simulink model "Isooffboard_SSC"  (R2026a)
settings: Solver=VariableStepAuto  StopTime=0.05
undefined symbols (not defined in the file): V_ref_isolated
libraries: fl_lib x73, nesl_utility x29, ee_lib x9, simulink x3, eeTransforms x2, batteryecm_lib x1, eeSinusoidalMeasurementV2 x1
(part 1 of 2)
settings Model: SimulationMode=accelerator  Creator=a6039  LastModifiedBy=agarcian
settings SimscapeCC: SimscapeNominalValues="[{\"value\":\"1\",\"unit\":\"A\"},{\"value\":\"1\",\"unit\":\"bar\"},{\"value\":\"1\",\"unit\":\"cm^2\"},{\"value\":\"1\",\"unit\":\"cm^3/s\"},{\"value\":\"1\",\"unit\":\"kJ/kg\"},{\"value\":\"1\",\"unit\":\"kW\"},{\"value\":\"1\",\"unit\":\"l\"},{\"value\":\"1\",\"unit\":\"N\"},{\"value\":\"1\",\"unit\":\"N*m\"},{\"value\":\"1\",\"unit\":\"V\"}]"  SimscapeLogType=none  SimscapeLogDataHistory=5000.0

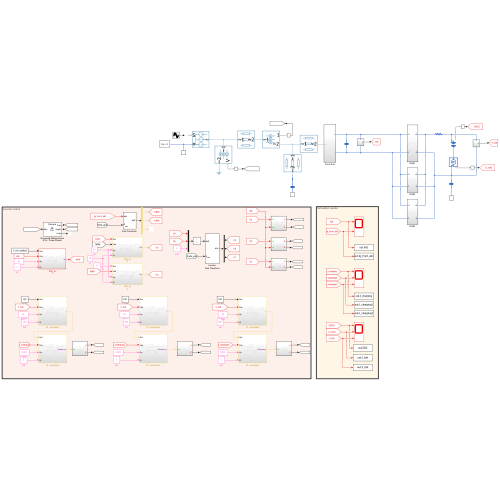
[thumbnail: Simulink's stored preview of the top-level diagram]
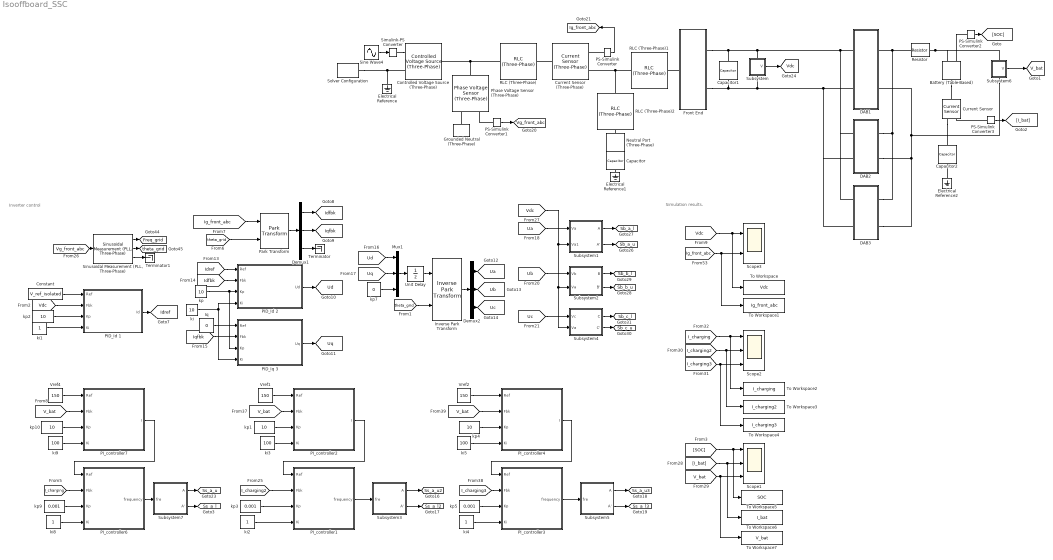
== system Isooffboard_SSC ==
  note: Simulation results.
  note: Inverter control
  Battery (Table-Based) : batteryecm_lib/Battery (Table-Based)  SOC_vec=[0, .1, .25, .5, .75, .9, 1]  T_dependence=simscape.enum.tablebattery.temperature_dependence.yes  prm_dir=simscape.enum.tablebattery.prm_dir.noCurrentDirectionality  T_vec=[278, 293, 313] K  V0_mat=[3.49, 3.5, 3.51; 3.55, 3.57, 3.56; 3.62, 3.63, 3.64; 3.71, 3.71, 3.72; 3.91, 3.93, 3.94; 4.07, 4.08, 4.08; 4.19, 4.19, 4.19] V  V0_vec=[3.5057, 3.566, 3.6337, 3.7127, 3.9259, 4.0777, 4.1928] V  V_range=[0, inf] V  R0_mat=[.0117, .0085, .009; .011, .0085, .009; .0114, .0087, .0092; .0107, .0082, .0088; .0107, .0083, .0091; .0113, .0085, .0089; .0116, .0085, .0089] Ohm  R0_vec=[.0085, .0085, .0087, .0082, .0083, .0085, .0085] Ohm  R0_dis_mat=[.0117, .0085, .009; .011, .0085, .009; .0114, .0087, .0092; .0107, .0082, .0088; .0107, .0083, .0091; .0113, .0085, .0089; .0116, .0085, .0089] Ohm  R0_dis_vec=[.0085, .0085, .0087, .0082, .0083, .0085, .0085] Ohm  R0_ch_mat=[.0117, .0085, .009; .011, .0085, .009; .0114, .0087, .0092; .0107, .0082, .0088; .0107, .0083, .0091; .0113, .0085, .0089; .0116, .0085, .0089] Ohm  R0_ch_vec=[.0085, .0085, .0087, .0082, .0083, .0085, .0085] Ohm  AH=5.4 A*hr  prm_leak=simscape.enum.tablebattery.prm_leak.disabled  Rleak_vec=[8000, 7000, 6000] Ohm  Rleak=7e3 Ohm  extrapolation_option=simscape.enum.extrapolation.nearest  SOC_port=simscape.enum.tablebattery.enable.yes  prm_dyn=simscape.enum.tablebattery.prm_dyn.off  R1_mat=[.0109, .0029, .0013; .0069, .0024, .0012; .0047, .0026, .0013; .0034, .0016, .001; .0033, .0023, .0014; .0033, .0018, .0011; .0028, .0017, .0011] Ohm  R1_vec=[.0029, .0024, .0026, .0016, .0023, .0018, .0017] Ohm  tau1_mat=[20, 36, 39; 31, 45, 39; 109, 105, 61; 36, 29, 26; 59, 77, 67; 40, 33, 29; 25, 39, 33] s  tau1_vec=[36, 45, 105, 29, 77, 33, 39] s  R2_mat=[.0109, .0029, .0013; .0069, .0024, .0012; .0047, .0026, .0013; .0034, .0016, .001; .0033, .0023, .0014; .0033, .0018, .0011; .0028, .0017, .0011] Ohm  R2_vec=[.0029, .0024, .0026, .0016, .0023, .0018, .0017] Ohm  tau2_mat=[20, 36, 39; 31, 45, 39; 109, 105, 61; 36, 29, 26; 59, 77, 67; 40, 33, 29; 25, 39, 33] s  tau2_vec=[36, 45, 105, 29, 77, 33, 39] s  R3_mat=[.0109, .0029, .0013; .0069, .0024, .0012; .0047, .0026, .0013; .0034, .0016, .001; .0033, .0023, .0014; .0033, .0018, .0011; .0028, .0017, .0011] Ohm  R3_vec=[.0029, .0024, .0026, .0016, .0023, .0018, .0017] Ohm  tau3_mat=[20, 36, 39; 31, 45, 39; 109, 105, 61; 36, 29, 26; 59, 77, 67; 40, 33, 29; 25, 39, 33] s  tau3_vec=[36, 45, 105, 29, 77, 33, 39] s  R4_mat=[.0109, .0029, .0013; .0069, .0024, .0012; .0047, .0026, .0013; .0034, .0016, .001; .0033, .0023, .0014; .0033, .0018, .0011; .0028, .0017, .0011] Ohm  R4_vec=[.0029, .0024, .0026, .0016, .0023, .0018, .0017] Ohm  tau4_mat=[20, 36, 39; 31, 45, 39; 109, 105, 61; 36, 29, 26; 59, 77, 67; 40, 33, 29; 25, 39, 33] s  tau4_vec=[36, 45, 105, 29, 77, 33, 39] s  R5_mat=[.0109, .0029, .0013; .0069, .0024, .0012; .0047, .0026, .0013; .0034, .0016, .001; .0033, .0023, .0014; .0033, .0018, .0011; .0028, .0017, .0011] Ohm  R5_vec=[.0029, .0024, .0026, .0016, .0023, .0018, .0017] Ohm  tau5_mat=[20, 36, 39; 31, 45, 39; 109, 105, 61; 36, 29, 26; 59, 77, 67; 40, 33, 29; 25, 39, 33] s  tau5_vec=[36, 45, 105, 29, 77, 33, 39] s  prm_fade=simscape.enum.tablebattery.prm_fade.disabled  N0=100  dV0=0  dR0=0  dAH=0  dRleak=0  dR1=0  dR2=0  dR3=0  dR4=0  dR5=0  N0vec=[0, 100, 200, 300]  Tfadevec=[298.15, 323.15] K  dV0vec=[0, 0, 0, 0]  dR0vec=[0, 0, 0, 0]  dAHvec=[0, 0, 0, 0]  dRleakvec=[0, 0, 0, 0]  dR1vec=[0, 0, 0, 0]  dR2vec=[0, 0, 0, 0]  dR3vec=[0, 0, 0, 0]  dR4vec=[0, 0, 0, 0]  dR5vec=[0, 0, 0, 0]  dV0mat=[0, 0; 0, 0; 0, 0; 0, 0]  dR0mat=[0, 0; 0, 0; 0, 0; 0, 0]  dAHmat=[0, 0; 0, 0; 0, 0; 0, 0]  dRleakmat=[0, 0; 0, 0; 0, 0; 0, 0]  dR1mat=[0, 0; 0, 0; 0, 0; 0, 0]  dR2mat=[0, 0; 0, 0; 0, 0; 0, 0]  dR3mat=[0, 0; 0, 0; 0, 0; 0, 0]  dR4mat=[0, 0; 0, 0; 0, 0; 0, 0]  dR5mat=[0, 0; 0, 0; 0, 0; 0, 0]  prm_age_modeling=simscape.enum.tablebattery.prm_age_modeling.equation  storage_dt_age_vec=[0] d  storage_T_age_vec=[273] K  prm_age_OCV=simscape.enum.tablebattery.prm_age_OCV.OCV  OCV_age=0.9  SOC_age=0.6  prm_age_resistance=simscape.enum.tablebattery.prm_age.disabled  OCV_scaling_age_resistance=2.2134e6  OCV_offset_age_resistance=1.632e6  temp_exp_age_resistance=0.515833569 V  t_exp_age_resistance=0.75  T_age_vec_resistance=[273.15, 298.15, 323.15] K  dt_age_vec_resistance=[0, 90, 180, 270] d  dR0_age_vec=[0, 0, 0]  t_meas_dR0_age=100 d  dR0_age_mat=[0, 0, 0; 0, 0, 0; 0, 0, 0; 0, 0, 0]  prm_age_capacity=simscape.enum.tablebattery.prm_age.disabled  OCV_scaling_age_capacity=1.5097e07  OCV_offset_age_capacity=8.3625e06  temp_exp_age_capacity=0.6011 V  t_exp_age_capacity=0.75  T_age_vec_capacity=[273.15, 298.15, 323.15] K  dt_age_vec_capacity=[0, 90, 180, 270] d  dAH_age_vec=[0, 0, 0]  t_meas_dAH_age=100 d  dAH_age_mat=[0, 0, 0; 0, 0, 0; 0, 0, 0; 0, 0, 0]  thermal_port=simscape.enum.thermaleffects.omit  temperature=298.15 K  thermal_mass=100 J/K  i_specify=off  i_priority=None  i=0 A  i_nominal_specify=off  i_nominal_value=1  i_nominal_unit=A  v_specify=off  v_priority=None  v=0 V  v_nominal_specify=off  v_nominal_value=1  v_nominal_unit=V  stateOfCharge_specify=off  stateOfCharge_priority=High  stateOfCharge=1  stateOfCharge_nominal_specify=off  stateOfCharge_nominal_value=1  stateOfCharge_nominal_unit=1  num_cycles_specify=off  num_cycles_priority=High  num_cycles=0  num_cycles_nominal_specify=off  num_cycles_nominal_value=1  num_cycles_nominal_unit=1  cell_temperature_specify=off  cell_temperature_priority=High  cell_temperature=298.15 K  cell_temperature_nominal_specify=off  cell_temperature_nominal_value=1  cell_temperature_nominal_unit=K
  Capacitor : fl_lib/Electrical/Electrical Elements/Capacitor  c=1e-8 F  r=0 Ohm  g=0 1/Ohm  i_specify=off  i_priority=None  i=0 A  i_nominal_specify=off  i_nominal_value=1  i_nominal_unit=A  v_specify=off  v_priority=None  v=0 V  v_nominal_specify=off  v_nominal_value=1  v_nominal_unit=V  vc_specify=off  vc_priority=High  vc=0 V  vc_nominal_specify=off  vc_nominal_value=1  vc_nominal_unit=V
  Capacitor1 : fl_lib/Electrical/Electrical Elements/Capacitor  c=500e-5 F  r=1e-9 Ohm  g=0 1/Ohm  i_specify=off  i_priority=None  i=0 A  i_nominal_specify=off  i_nominal_value=1  i_nominal_unit=A  v_specify=off  v_priority=None  v=0 V  v_nominal_specify=off  v_nominal_value=1  v_nominal_unit=V  vc_specify=off  vc_priority=High  vc=0 V  vc_nominal_specify=off  vc_nominal_value=1  vc_nominal_unit=V
  Capacitor2 : fl_lib/Electrical/Electrical Elements/Capacitor  c=1e-9 F  r=0 Ohm  g=0 1/Ohm  i_specify=off  i_priority=None  i=0 A  i_nominal_specify=off  i_nominal_value=1  i_nominal_unit=A  v_specify=off  v_priority=None  v=0 V  v_nominal_specify=off  v_nominal_value=1  v_nominal_unit=V  vc_specify=off  vc_priority=High  vc=0 V  vc_nominal_specify=off  vc_nominal_value=1  vc_nominal_unit=V
  Constant : Constant  Value=V_ref_isolated
  Controlled Voltage Source (Three-Phase) : ee_lib/Sources/Controlled Voltage Source (Three-Phase)  input_option=ee.enum.inputType.instantaneous  FRated=60 Hz
  Current Sensor : fl_lib/Electrical/Electrical Sensors/Current Sensor
  Current Sensor (Three-Phase) : ee_lib/Sensors & Transducers/Current Sensor (Three-Phase)  port_option=ee.enum.threePhasePort.composite
  DAB1 : Subsystem
  DAB2 : Subsystem
  DAB3 : Subsystem
  Demux1 : Demux  Outputs=3
  Demux2 : Demux  Outputs=3
  Electrical Reference : fl_lib/Electrical/Electrical Elements/Electrical Reference
  Electrical Reference1 : fl_lib/Electrical/Electrical Elements/Electrical Reference
  Electrical Reference2 : fl_lib/Electrical/Electrical Elements/Electrical Reference
  Front End : Subsystem
  Grounded Neutral (Three-Phase) : ee_lib/Connectors & References/Grounded Neutral (Three-Phase)  port_option=ee.enum.threePhasePort.composite
  Inverse Park Transform : eeTransforms/Inverse Park Transform  AxisAlignment=Q-axis  PowerInvariant=off
      settings: LibrarySourceBlock=|
      | ee_sl_lib/Mathematical
      | Transforms/Inverse
      | Park Transform
  Iq : Constant  Value=0
  Mux1 : Mux  Inputs=3
  Neutral Port (Three-Phase) : ee_lib/Connectors & References/Neutral Port (Three-Phase)  port_option=ee.enum.threePhasePort.composite  G_parasitic=1e-12 1/Ohm
  PID_Id 1 : Subsystem
  PID_Id 2 : Subsystem
  PID_Iq 3 : Subsystem
  PI_controller1 : Subsystem
  PI_controller2 : Subsystem
  PI_controller3 : Subsystem
  PI_controller4 : Subsystem
  PI_controller6 : Subsystem
  PI_controller7 : Subsystem
  PS-Simulink Converter{,1..3} (4 alike) : nesl_utility/PS-Simulink Converter  PhysicalDomain=network_engine_domain  SubClassName=ps_output  LeftPortType=input  RightPortType=output  PseudoPeriodic=off  Frequencies=[]  VectorFormat=inherit  Unit=inherit  AffineConversion=off
  Park Transform : eeTransforms/Park Transform  AxisAlignment=Q-axis  PowerInvariant=off
      settings: LibrarySourceBlock=|
      | ee_sl_lib/Mathematical
      | Transforms/Park Transform
  Phase Voltage Sensor (Three-Phase) : ee_lib/Sensors & Transducers/Phase Voltage Sensor (Three-Phase)  port_option=ee.enum.threePhasePort.composite
  RLC (Three-Phase) : ee_lib/Passive/RLC Assemblies/RLC (Three-Phase)  port_option=ee.enum.threePhasePort.composite  component_structure=ee.enum.rlc.structure.SeriesRL  R=1 Ohm  L=1e-9 H  C=1e-6 F  R_parasitic=0 Ohm  G_parasitic=0 1/Ohm  IL_specify=off  IL_priority=High  IL=[0, 0, 0] A  IL_nominal_specify=off  IL_nominal_value=1  IL_nominal_unit=A  VC_specify=off  VC_priority=High  VC=[0, 0, 0] V  VC_nominal_specify=off  VC_nominal_value=1  VC_nominal_unit=V
  RLC (Three-Phase)1 : ee_lib/Passive/RLC Assemblies/RLC (Three-Phase)  port_option=ee.enum.threePhasePort.composite  component_structure=ee.enum.rlc.structure.SeriesRL  R=0.1 Ohm  L=80e-6 H  C=1e-6 F  R_parasitic=0 Ohm  G_parasitic=0 1/Ohm  IL_specify=off  IL_priority=High  IL=[0, 0, 0] A  IL_nominal_specify=off  IL_nominal_value=1  IL_nominal_unit=A  VC_specify=off  VC_priority=High  VC=[0, 0, 0] V  VC_nominal_specify=off  VC_nominal_value=1  VC_nominal_unit=V
  RLC (Three-Phase)2 : ee_lib/Passive/RLC Assemblies/RLC (Three-Phase)  port_option=ee.enum.threePhasePort.composite  component_structure=ee.enum.rlc.structure.SeriesRC  R=1e-9 Ohm  L=80e-6 H  C=80e-5 F  R_parasitic=0 Ohm  G_parasitic=0 1/Ohm  IL_specify=off  IL_priority=High  IL=[0, 0, 0] A  IL_nominal_specify=off  IL_nominal_value=1  IL_nominal_unit=A  VC_specify=off  VC_priority=High  VC=[0, 0, 0] V  VC_nominal_specify=off  VC_nominal_value=1  VC_nominal_unit=V
  Resistor : fl_lib/Electrical/Electrical Elements/Resistor  R=1e-5 Ohm  i_specify=off  i_priority=None  i=0 A  i_nominal_specify=off  i_nominal_value=1  i_nominal_unit=A  v_specify=off  v_priority=None  v=0 V  v_nominal_specify=off  v_nominal_value=1  v_nominal_unit=V
  Scope1 : Scope  NumInputPorts=3
      settings: ActiveDisplayYMinimum=1.0000206621437779  ActiveDisplayYMaximum=1.0000384781316543
  Scope2 : Scope  NumInputPorts=3
      settings: ActiveDisplayYMinimum=-219.29902  ActiveDisplayYMaximum=119.1691  DataLoggingVariableName=ScopeData2
  Scope3 : Scope  NumInputPorts=2
      settings: ActiveDisplayYMinimum=-113.39678269473124  ActiveDisplayYMaximum=1020.5710233769659
  Simulink-PS Converter : nesl_utility/Simulink-PS Converter  PhysicalDomain=network_engine_domain  SubClassName=ps_input  LeftPortType=input  RightPortType=output  PseudoPeriodic=off  Frequencies=[]  NoiseDistribution=none  NoiseParameters=[]  Unit=1  AffineConversion=off  FilteringAndDerivatives=provide  SimscapeFilterOrder=1  InputFilterTimeConstant=0.001  UdotUserProvided=0
  Sine Wave4 : Sin  Amplitude=480  Frequency=60*2*pi  Phase=[0 -1 1]*2*pi/3  SampleTime=1e-7
  "Sinusoidal Measurement (PLL, Three-Phase)" : eeSinusoidalMeasurementV2/Sinusoidal Measurement (PLL, Three-Phase)  InputFilter=on  InputNormalization=off  Kp_LF=180  Ki_LF=3200  F0=60  Theta0=0  Ts=0.0001
      settings: LibrarySourceBlock=|
      | ee_sl_lib/Measurements/Sinusoidal Measurement
      | (PLL, Three-Phase)
  Solver Configuration : nesl_utility/Solver Configuration  PhysicalDomain=network_engine_domain  SubClassName=solver  LeftPortType=input  RightPortType=generic  Tones=[]  Harmonics=[]  SimulateNoise=off  Profile=off  UseLocalSampling=off  EnableSwitchedLinearOptims=on  FrequencyDomain=off  UseCCode=off  RelTol=0.001  AbsTol=0.001  MinStep=1e-09  ToWorkspace=off  RevertToSquareIcSolve=off  NumHomotopyIterations=100  PhasorMode=off  PhasorModeNumHarmonics=1  ConsistencySolver=NEWTON_XTOL_AFTER_FTOL  CanonicalOrdering=UNORDERED  OptimizeIntermediates=UNOPTIMIZED  IndexReductionMethod=DerivativeReplacement  DoDC=off  ResidualTolerance=1e-09  ConsistencyTolSource=GLOBAL  ConsistencyAbsTol=0.001  ConsistencyRelTol=0.001  ConsistencyTolFactor=0.001  UseLocalSolver=on  LocalSolverChoice=NE_PARTITIONING_ADVANCER  ResolveIndetEquations=off  FunctionEvalNumThread=1  LocalSolverSampleTime=1e-7  DoFixedCost=off  MaxNonlinIter=2  MaxModeIter=2  ComputeImpulses=off  ImpulseIterations=2  LinearAlgebra=auto  LinearAlgebraNumThread=0  EquationFormulation=NE_TIME_EF  DelaysMemoryBudget=1024  AutomaticFiltering=off  FilteringTimeConstant=0.001  PartitionStorageMethod=AS_NEEDED  PartitionMemoryBudget=1024  PartitionMethod=ROBUST  MultibodyUseLocalSolver=off  MultibodyLocalSolverChoice=ODE1  MultibodyLocalSolverSampleTime=0.001
  Subsystem : Subsystem
      settings: PortSchema="{\"entries\":[{\"content\":{\"sides\":[{\"content\":{},\"type\":\"ConnectorPlacement.EquallySpacedRectSide\",\"uuid\":\"5292a83f-6f3d-4481-9274-991c3d86e7c3\"},{\"content\":{\"connectorIds\":[\"Out1\"],\"side\":\"RIGHT\"},\"type\":\"ConnectorPlacement.EquallySpacedRectSide\",\"uuid\":\"3f03e0e6-bee9-49df-bbfb-7f0a1aca1df7\"},{\"content\":{\"connectorIds\":[\"LConn1\"],\"side\":\"TOP\"},\"type\":\"ConnectorPlacement.EquallySpacedRectSide\",\"uuid\":\"842fbd6d-a974-4b26-821b-48593ae4fc83\"},{\"content\":{\"connectorIds\":[\"RConn1\"],\"side\":\"BOTTOM\"},\"type\":\"ConnectorPlacement.EquallySpacedRectSide\",\"uuid\":\"ab18bb4b-4bc5-4d22-a9fd-5b5abd0ee64f\"}]},\"type\":\"ConnectorPlacement.EquallySpacedConnector\",\"uuid\":\"a2f9b0d8-8bc3-4cf1-85b9-fb5408ef68da\"}],\"packageUris\":[\"http://schema.mathworks.com/mf0/Connector/R2020b\"],\"version\":\"1.0\"}"
  Subsystem1 : Subsystem
  Subsystem2 : Subsystem
  Subsystem3 : Subsystem
  Subsystem4 : Subsystem
  Subsystem5 : Subsystem
  Subsystem6 : Subsystem
      settings: PortSchema="{\"entries\":[{\"content\":{\"sides\":[{\"content\":{},\"type\":\"ConnectorPlacement.EquallySpacedRectSide\",\"uuid\":\"5292a83f-6f3d-4481-9274-991c3d86e7c3\"},{\"content\":{\"connectorIds\":[\"Out1\"],\"side\":\"RIGHT\"},\"type\":\"ConnectorPlacement.EquallySpacedRectSide\",\"uuid\":\"3f03e0e6-bee9-49df-bbfb-7f0a1aca1df7\"},{\"content\":{\"connectorIds\":[\"LConn1\"],\"side\":\"TOP\"},\"type\":\"ConnectorPlacement.EquallySpacedRectSide\",\"uuid\":\"842fbd6d-a974-4b26-821b-48593ae4fc83\"},{\"content\":{\"connectorIds\":[\"RConn1\"],\"side\":\"BOTTOM\"},\"type\":\"ConnectorPlacement.EquallySpacedRectSide\",\"uuid\":\"ab18bb4b-4bc5-4d22-a9fd-5b5abd0ee64f\"}]},\"type\":\"ConnectorPlacement.EquallySpacedConnector\",\"uuid\":\"a2f9b0d8-8bc3-4cf1-85b9-fb5408ef68da\"}],\"packageUris\":[\"http://schema.mathworks.com/mf0/Connector/R2020b\"],\"version\":\"1.0\"}"
  Subsystem7 : Subsystem
  Terminator : Terminator
  Terminator1 : Terminator
  To Workspace : ToWorkspace  VariableName=Vdc  SaveFormat=Structure With Time  SampleTime=-1
      settings: Decimation=100
  To Workspace1 : ToWorkspace  VariableName=Ig_front_abc  SaveFormat=Structure With Time  SampleTime=-1
  To Workspace2 : ToWorkspace  VariableName=I_charging  SaveFormat=Structure With Time  SampleTime=-1
      settings: Decimation=100
  To Workspace3 : ToWorkspace  VariableName=I_charging2  SaveFormat=Structure With Time  SampleTime=-1
      settings: Decimation=100
  To Workspace4 : ToWorkspace  VariableName=I_charging3  SampleTime=-1
      settings: Decimation=100
  To Workspace5 : ToWorkspace  VariableName=SOC  SaveFormat=Structure With Time  SampleTime=-1
      settings: Decimation=100
  To Workspace6 : ToWorkspace  VariableName=I_bat  SaveFormat=Structure With Time  SampleTime=-1
      settings: Decimation=100
  To Workspace7 : ToWorkspace  VariableName=V_bat  SaveFormat=Structure With Time  SampleTime=-1
      settings: Decimation=100
  Unit Delay : UnitDelay  SampleTime=-1
  Vref1 : Constant  Value=150
  Vref2 : Constant  Value=150
  Vref4 : Constant  Value=150
  ki : Constant  Value=10
  ki{1..2,4,8} (4 alike) : Constant
  ki3 : Constant  Value=100
  ki5 : Constant  Value=100
  ki9 : Constant  Value=100
  kp{,1..2,4,10} (5 alike) : Constant  Value=10
  kp3 : Constant  Value=0.001
  kp5 : Constant  Value=0.001
  kp7 : Constant  Value=0
  kp9 : Constant  Value=0.001
  tag scope: Freq_grid=global, Idfbk=global, Idref=global, Ig_front_abc=global, Iqfbk=global, Sb_a_l=global, Sb_a_u=global, Sb_b_l=global, Sb_b_u=global, Sb_c_l=global, Sb_c_u=global, Ss_a_l2=global, Ss_a_l3=global, Ss_a_l=global, Ss_a_u2=global, Ss_a_u3=global, Ss_a_u=global, Ua=global, Ub=global, Uc=global, Ud=global, Uq=global, V_bat=global, Vdc=global, Vg_front_abc=global, theta_grid=global
  wires:
  Mux1/1 -> Unit Delay/1
  Demux2/3 -> [Uc]
  ki1/1 -> PID_Id 1/4(Ki)
  Demux2/1 -> [Ua]
  [theta_grid] -> Inverse Park Transform/2
  Demux2/2 -> [Ub]
  [Uq] -> Mux1/2
  [Ua] -> Subsystem1/1(Va)
  Demux1/2 -> [Iqfbk]
  [Idfbk] -> PID_Id 2/2(Fbk)
  [Idref] -> PID_Id 2/1(Ref)
  Demux1/1 -> [Idfbk]
  PID_Id 1/1(Id) -> [Idref]
  kp7/1 -> Mux1/3
  PID_Id 2/1(Ud) -> [Ud]
  PID_Iq 3/1(Uq) -> [Uq]
  [Ud] -> Mux1/1
  [Uc] -> Subsystem4/1(Vc)
  [Iqfbk] -> PID_Iq 3/2(Fbk)
  [Vdc] -> PID_Id 1/2(Fbk)
  Constant/1 -> PID_Id 1/1(Ref)
  ki/1 -> PID_Iq 3/4(Ki), PID_Id 2/4(Ki)
  [Ig_front_abc] -> Park Transform/1
  [Ub] -> Subsystem2/1(Vb)
  Iq/1 -> PID_Iq 3/1(Ref)
  Inverse Park Transform/1 -> Demux2/1
  Park Transform/1 -> Demux1/1
  kp/1 -> PID_Iq 3/3(Kp), PID_Id 2/3(Kp)
  [theta_grid] -> Park Transform/2
  kp2/1 -> PID_Id 1/3(Kp)
  Subsystem1/2(A') -> [Sb_a_u]
  Subsystem1/1(A) -> [Sb_a_l]
  Subsystem2/2(B') -> [Sb_b_u]
  Subsystem2/1(B) -> [Sb_b_l]
  Subsystem4/2(C') -> [Sb_c_u]
  Subsystem4/1(C) -> [Sb_c_l]
  [Ig_front_abc] -> To Workspace1/1, Scope3/2
  [Vdc] -> To Workspace/1, Scope3/1
  [Vg_front_abc] -> "Sinusoidal Measurement (PLL, Three-Phase)"/1
  "Sinusoidal Measurement (PLL, Three-Phase)"/1 -> [Freq_grid]
  "Sinusoidal Measurement (PLL, Three-Phase)"/2 -> [theta_grid]
  [Vdc] -> Subsystem4/2(Va), Subsystem2/2(Va), Subsystem1/2(Va1)
  [I_bat] -> Scope1/2, To Workspace6/1
  [V_bat] -> Scope1/3, To Workspace7/1
  [I_charging] -> To Workspace2/1, Scope2/1
  [I_charging2] -> To Workspace3/1, Scope2/2
  [I_charging3] -> To Workspace4/1, Scope2/3
  ki9/1 -> PI_controller7/4(Ki)
  PI_controller6/1(frequency) -> Subsystem7/1(fre)
  [V_bat] -> PI_controller7/2(Fbk)
  [I_charging] -> PI_controller6/2(Fbk)
  Subsystem7/2(A') -> [Ss_a_l]
  PI_controller7/1(I) -> PI_controller6/1(Ref)
  ki8/1 -> PI_controller6/4(Ki)
  Vref4/1 -> PI_controller7/1(Ref)
  Subsystem7/1(A) -> [Ss_a_u]
  kp9/1 -> PI_controller6/3(Kp)
  kp10/1 -> PI_controller7/3(Kp)
  kp3/1 -> PI_controller1/3(Kp)
  ki3/1 -> PI_controller2/4(Ki)
  Subsystem3/2(A') -> [Ss_a_l2]
  Subsystem3/1(A) -> [Ss_a_u2]
  PI_controller1/1(frequency) -> Subsystem3/1(fre)
  Vref1/1 -> PI_controller2/1(Ref)
  [I_charging2] -> PI_controller1/2(Fbk)
  ki2/1 -> PI_controller1/4(Ki)
  [V_bat] -> PI_controller2/2(Fbk)
  kp1/1 -> PI_controller2/3(Kp)
  PI_controller2/1(I) -> PI_controller1/1(Ref)
  PI_controller4/1(I) -> PI_controller3/1(Ref)
  kp4/1 -> PI_controller4/3(Kp)
  ki4/1 -> PI_controller3/4(Ki)
  [V_bat] -> PI_controller4/2(Fbk)
  Vref2/1 -> PI_controller4/1(Ref)
  PI_controller3/1(frequency) -> Subsystem5/1(fre)
  ki5/1 -> PI_controller4/4(Ki)
  Subsystem5/1(A) -> [Ss_a_u3]
  [I_charging3] -> PI_controller3/2(Fbk)
  Subsystem5/2(A') -> [Ss_a_l3]
  kp5/1 -> PI_controller3/3(Kp)
  PS-Simulink Converter1/1 -> [Vg_front_abc]
  PS-Simulink Converter/1 -> [Ig_front_abc]
  Sine Wave4/1 -> Simulink-PS Converter/1
  Unit Delay/1 -> Inverse Park Transform/1
  Demux1/3 -> Terminator/1
  Subsystem/1(V) -> [Vdc]
  Subsystem6/1(V) -> [V_bat]
  "Sinusoidal Measurement (PLL, Three-Phase)"/3 -> Terminator1/1
  PS-Simulink Converter2/1 -> [SOC]
  PS-Simulink Converter3/1 -> [I_bat]
  [SOC] -> Scope1/1, To Workspace5/1
  connections:
  Electrical Reference/LConn1 -- Solver Configuration/RConn1 -- Controlled Voltage Source (Three-Phase)/LConn2
  RLC (Three-Phase)/LConn1 -- Phase Voltage Sensor (Three-Phase)/LConn1 -- Controlled Voltage Source (Three-Phase)/RConn1
  Grounded Neutral (Three-Phase)/LConn1 -- Phase Voltage Sensor (Three-Phase)/RConn2
  Current Sensor (Three-Phase)/LConn1 -- RLC (Three-Phase)/RConn1
  RLC (Three-Phase)1/LConn1 -- Current Sensor (Three-Phase)/RConn2 -- RLC (Three-Phase)2/LConn1
  PS-Simulink Converter/LConn1 -- Current Sensor (Three-Phase)/RConn1
  PS-Simulink Converter1/LConn1 -- Phase Voltage Sensor (Three-Phase)/RConn1
  Neutral Port (Three-Phase)/LConn1 -- RLC (Three-Phase)2/RConn1
  Capacitor/LConn1 -- Neutral Port (Three-Phase)/RConn1
  Electrical Reference1/LConn1 -- Capacitor/RConn1
  Front End/LConn1 -- RLC (Three-Phase)1/RConn1
  Capacitor1/RConn1 -- Front End/RConn2 -- DAB3/LConn2 -- DAB2/LConn2 -- DAB1/LConn2 -- Subsystem/RConn1
  DAB2/RConn1 -- DAB3/RConn1 -- Resistor/LConn1 -- DAB1/RConn1
  DAB2/RConn2 -- Current Sensor/RConn2 -- Capacitor2/LConn1 -- Subsystem6/RConn1 -- DAB1/RConn2 -- DAB3/RConn2
  Simulink-PS Converter/RConn1 -- Controlled Voltage Source (Three-Phase)/LConn1
  Electrical Reference2/LConn1 -- Capacitor2/RConn1
  Resistor/RConn1 -- Battery (Table-Based)/LConn1 -- Subsystem6/LConn1
  Capacitor1/LConn1 -- Front End/RConn1 -- DAB3/LConn1 -- DAB2/LConn1 -- DAB1/LConn1 -- Subsystem/LConn1
  Battery (Table-Based)/LConn2 -- PS-Simulink Converter2/LConn1
  Battery (Table-Based)/RConn1 -- Current Sensor/LConn1
  PS-Simulink Converter3/LConn1 -- Current Sensor/RConn1

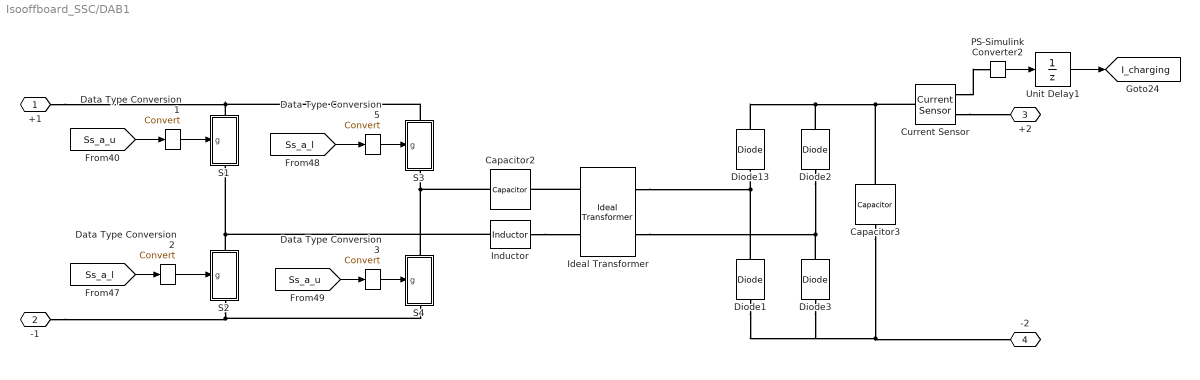
== system Isooffboard_SSC/DAB1 ==
  Capacitor2 : fl_lib/Electrical/Electrical Elements/Capacitor  c=110e-9 F  r=1e-6 Ohm  g=0 1/Ohm  i_specify=off  i_priority=None  i=0 A  i_nominal_specify=off  i_nominal_value=1  i_nominal_unit=A  v_specify=off  v_priority=None  v=0 V  v_nominal_specify=off  v_nominal_value=1  v_nominal_unit=V  vc_specify=off  vc_priority=High  vc=0 V  vc_nominal_specify=off  vc_nominal_value=1  vc_nominal_unit=V
  Capacitor3 : fl_lib/Electrical/Electrical Elements/Capacitor  c=500e-6 F  r=0 Ohm  g=0 1/Ohm  i_specify=off  i_priority=None  i=0 A  i_nominal_specify=off  i_nominal_value=1  i_nominal_unit=A  v_specify=off  v_priority=None  v=0 V  v_nominal_specify=off  v_nominal_value=1  v_nominal_unit=V  vc_specify=off  vc_priority=High  vc=0 V  vc_nominal_specify=off  vc_nominal_value=1  vc_nominal_unit=V
  Current Sensor : fl_lib/Electrical/Electrical Sensors/Current Sensor
  Data Type Conversion{1..3,5} (4 alike) : DataTypeConversion  SaturateOnIntegerOverflow=off  RndMeth=Floor
  Diode{1..3,13} (4 alike) : fl_lib/Electrical/Electrical Elements/Diode  Vf=0.8 V  Ron=0.001 Ohm  Goff=1/500 1/Ohm  i_specify=off  i_priority=None  i=0 A  i_nominal_specify=off  i_nominal_value=1  i_nominal_unit=A  v_specify=off  v_priority=None  v=0 V  v_nominal_specify=off  v_nominal_value=1  v_nominal_unit=V
  Ideal Transformer : fl_lib/Electrical/Electrical Elements/Ideal Transformer  n=1  i1_specify=off  i1_priority=None  i1=0 A  i1_nominal_specify=off  i1_nominal_value=1  i1_nominal_unit=A  v1_specify=off  v1_priority=None  v1=0 V  v1_nominal_specify=off  v1_nominal_value=1  v1_nominal_unit=V  i2_specify=off  i2_priority=None  i2=0 A  i2_nominal_specify=off  i2_nominal_value=1  i2_nominal_unit=A  v2_specify=off  v2_priority=None  v2=0 V  v2_nominal_specify=off  v2_nominal_value=1  v2_nominal_unit=V
  Inductor : fl_lib/Electrical/Electrical Elements/Inductor  l=21e-6 H  r=1e-6 Ohm  g=0 1/Ohm  i_specify=off  i_priority=None  i=0 A  i_nominal_specify=off  i_nominal_value=1  i_nominal_unit=A  v_specify=off  v_priority=None  v=0 V  v_nominal_specify=off  v_nominal_value=1  v_nominal_unit=V  i_L_specify=off  i_L_priority=High  i_L=0 A  i_L_nominal_specify=off  i_L_nominal_value=1  i_L_nominal_unit=A
  PS-Simulink Converter2 : nesl_utility/PS-Simulink Converter  PhysicalDomain=network_engine_domain  SubClassName=ps_output  LeftPortType=input  RightPortType=output  PseudoPeriodic=off  Frequencies=[]  VectorFormat=inherit  Unit=inherit  AffineConversion=off
  S1 : Subsystem
      settings: PortSchema="{\"entries\":[{\"content\":{\"sides\":[{\"content\":{\"connectorIds\":[\"In1\"]},\"type\":\"ConnectorPlacement.EquallySpacedRectSide\",\"uuid\":\"4868c43b-8f86-4e2f-a4da-367c2e17d6e4\"},{\"content\":{\"side\":\"RIGHT\"},\"type\":\"ConnectorPlacement.EquallySpacedRectSide\",\"uuid\":\"ebe9b5ec-833b-4a08-98e5-ff684cd7afcb\"},{\"content\":{\"connectorIds\":[\"LConn1\"],\"side\":\"TOP\"},\"type\":\"ConnectorPlacement.EquallySpacedRectSide\",\"uuid\":\"c72df866-8baa-41a8-9bb1-42a4a1fdee71\"},{\"content\":{\"connectorIds\":[\"RConn1\"],\"side\":\"BOTTOM\"},\"type\":\"ConnectorPlacement.EquallySpacedRectSide\",\"uuid\":\"3a9867c5-1563-48cb-a4f4-92deec85fd3d\"}]},\"type\":\"ConnectorPlacement.EquallySpacedConnector\",\"uuid\":\"206e0d7b-1d35-45e7-9c4c-8a6f9fe9dc79\"}],\"packageUris\":[\"http://schema.mathworks.com/mf0/Connector/R2020b\"],\"version\":\"1.0\"}"
  S2 : Subsystem
      settings: PortSchema="{\"entries\":[{\"content\":{\"sides\":[{\"content\":{\"connectorIds\":[\"In1\"]},\"type\":\"ConnectorPlacement.EquallySpacedRectSide\",\"uuid\":\"4868c43b-8f86-4e2f-a4da-367c2e17d6e4\"},{\"content\":{\"side\":\"RIGHT\"},\"type\":\"ConnectorPlacement.EquallySpacedRectSide\",\"uuid\":\"ebe9b5ec-833b-4a08-98e5-ff684cd7afcb\"},{\"content\":{\"connectorIds\":[\"LConn1\"],\"side\":\"TOP\"},\"type\":\"ConnectorPlacement.EquallySpacedRectSide\",\"uuid\":\"c72df866-8baa-41a8-9bb1-42a4a1fdee71\"},{\"content\":{\"connectorIds\":[\"RConn1\"],\"side\":\"BOTTOM\"},\"type\":\"ConnectorPlacement.EquallySpacedRectSide\",\"uuid\":\"3a9867c5-1563-48cb-a4f4-92deec85fd3d\"}]},\"type\":\"ConnectorPlacement.EquallySpacedConnector\",\"uuid\":\"206e0d7b-1d35-45e7-9c4c-8a6f9fe9dc79\"}],\"packageUris\":[\"http://schema.mathworks.com/mf0/Connector/R2020b\"],\"version\":\"1.0\"}"
  S3 : Subsystem
      settings: PortSchema="{\"entries\":[{\"content\":{\"sides\":[{\"content\":{\"connectorIds\":[\"In1\"]},\"type\":\"ConnectorPlacement.EquallySpacedRectSide\",\"uuid\":\"4868c43b-8f86-4e2f-a4da-367c2e17d6e4\"},{\"content\":{\"side\":\"RIGHT\"},\"type\":\"ConnectorPlacement.EquallySpacedRectSide\",\"uuid\":\"ebe9b5ec-833b-4a08-98e5-ff684cd7afcb\"},{\"content\":{\"connectorIds\":[\"LConn1\"],\"side\":\"TOP\"},\"type\":\"ConnectorPlacement.EquallySpacedRectSide\",\"uuid\":\"c72df866-8baa-41a8-9bb1-42a4a1fdee71\"},{\"content\":{\"connectorIds\":[\"RConn1\"],\"side\":\"BOTTOM\"},\"type\":\"ConnectorPlacement.EquallySpacedRectSide\",\"uuid\":\"3a9867c5-1563-48cb-a4f4-92deec85fd3d\"}]},\"type\":\"ConnectorPlacement.EquallySpacedConnector\",\"uuid\":\"206e0d7b-1d35-45e7-9c4c-8a6f9fe9dc79\"}],\"packageUris\":[\"http://schema.mathworks.com/mf0/Connector/R2020b\"],\"version\":\"1.0\"}"
  S4 : Subsystem
      settings: PortSchema="{\"entries\":[{\"content\":{\"sides\":[{\"content\":{\"connectorIds\":[\"In1\"]},\"type\":\"ConnectorPlacement.EquallySpacedRectSide\",\"uuid\":\"4868c43b-8f86-4e2f-a4da-367c2e17d6e4\"},{\"content\":{\"side\":\"RIGHT\"},\"type\":\"ConnectorPlacement.EquallySpacedRectSide\",\"uuid\":\"ebe9b5ec-833b-4a08-98e5-ff684cd7afcb\"},{\"content\":{\"connectorIds\":[\"LConn1\"],\"side\":\"TOP\"},\"type\":\"ConnectorPlacement.EquallySpacedRectSide\",\"uuid\":\"c72df866-8baa-41a8-9bb1-42a4a1fdee71\"},{\"content\":{\"connectorIds\":[\"RConn1\"],\"side\":\"BOTTOM\"},\"type\":\"ConnectorPlacement.EquallySpacedRectSide\",\"uuid\":\"3a9867c5-1563-48cb-a4f4-92deec85fd3d\"}]},\"type\":\"ConnectorPlacement.EquallySpacedConnector\",\"uuid\":\"206e0d7b-1d35-45e7-9c4c-8a6f9fe9dc79\"}],\"packageUris\":[\"http://schema.mathworks.com/mf0/Connector/R2020b\"],\"version\":\"1.0\"}"
  Unit Delay1 : UnitDelay  SampleTime=-1
  +1 : PMIOPort  Side=Left
  -1 : PMIOPort  Port=2  Side=Left
  +2 : PMIOPort  Port=3  Side=Right
  -2 : PMIOPort  Port=4  Side=Right
  tag scope: I_charging=global
  wires:
  [Ss_a_l] -> Data Type Conversion2/1
  [Ss_a_l] -> Data Type Conversion5/1
  PS-Simulink Converter2/1 -> Unit Delay1/1
  [Ss_a_u] -> Data Type Conversion3/1
  [Ss_a_u] -> Data Type Conversion1/1
  Data Type Conversion5/1 -> S3/1(g)
  Data Type Conversion1/1 -> S1/1(g)
  Data Type Conversion2/1 -> S2/1(g)
  Data Type Conversion3/1 -> S4/1(g)
  Unit Delay1/1 -> [I_charging]
  connections:
  S2/LConn1 -- Inductor/LConn1 -- S1/RConn1
  Diode13/RConn1 -- Diode2/RConn1 -- Current Sensor/LConn1 -- Capacitor3/LConn1
  Inductor/RConn1 -- Ideal Transformer/LConn2
  Ideal Transformer/RConn2 -- Diode3/RConn1 -- Diode2/LConn1
  S1/LConn1 -- S3/LConn1 -- +1/RConn1
  S4/LConn1 -- Capacitor2/LConn1 -- S3/RConn1
  Diode3/LConn1 -- Diode1/LConn1 -- Capacitor3/RConn1 -- -2/RConn1
  Ideal Transformer/LConn1 -- Capacitor2/RConn1
  Current Sensor/RConn1 -- PS-Simulink Converter2/LConn1
  Ideal Transformer/RConn1 -- Diode1/RConn1 -- Diode13/LConn1
  S2/RConn1 -- -1/RConn1 -- S4/RConn1
  Current Sensor/RConn2 -- +2/RConn1

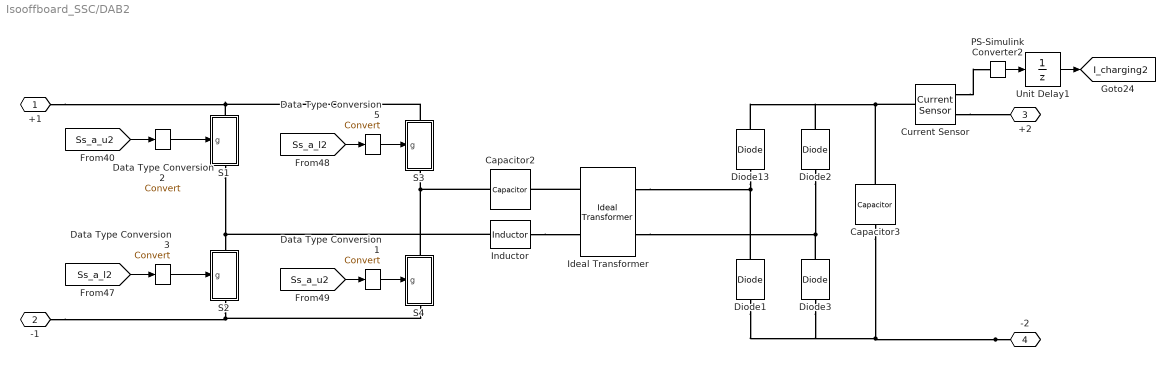
== system Isooffboard_SSC/DAB2 ==
  Capacitor2 : fl_lib/Electrical/Electrical Elements/Capacitor  c=110e-9 F  r=1e-6 Ohm  g=0 1/Ohm  i_specify=off  i_priority=None  i=0 A  i_nominal_specify=off  i_nominal_value=1  i_nominal_unit=A  v_specify=off  v_priority=None  v=0 V  v_nominal_specify=off  v_nominal_value=1  v_nominal_unit=V  vc_specify=off  vc_priority=High  vc=0 V  vc_nominal_specify=off  vc_nominal_value=1  vc_nominal_unit=V
  Capacitor3 : fl_lib/Electrical/Electrical Elements/Capacitor  c=500e-6 F  r=0 Ohm  g=0 1/Ohm  i_specify=off  i_priority=None  i=0 A  i_nominal_specify=off  i_nominal_value=1  i_nominal_unit=A  v_specify=off  v_priority=None  v=0 V  v_nominal_specify=off  v_nominal_value=1  v_nominal_unit=V  vc_specify=off  vc_priority=High  vc=0 V  vc_nominal_specify=off  vc_nominal_value=1  vc_nominal_unit=V
  Current Sensor : fl_lib/Electrical/Electrical Sensors/Current Sensor
  Data Type Conversion{1..3,5} (4 alike) : DataTypeConversion  SaturateOnIntegerOverflow=off  RndMeth=Floor
  Diode{1..3,13} (4 alike) : fl_lib/Electrical/Electrical Elements/Diode  Vf=0.8 V  Ron=0.001 Ohm  Goff=1/500 1/Ohm  i_specify=off  i_priority=None  i=0 A  i_nominal_specify=off  i_nominal_value=1  i_nominal_unit=A  v_specify=off  v_priority=None  v=0 V  v_nominal_specify=off  v_nominal_value=1  v_nominal_unit=V
  Ideal Transformer : fl_lib/Electrical/Electrical Elements/Ideal Transformer  n=1  i1_specify=off  i1_priority=None  i1=0 A  i1_nominal_specify=off  i1_nominal_value=1  i1_nominal_unit=A  v1_specify=off  v1_priority=None  v1=0 V  v1_nominal_specify=off  v1_nominal_value=1  v1_nominal_unit=V  i2_specify=off  i2_priority=None  i2=0 A  i2_nominal_specify=off  i2_nominal_value=1  i2_nominal_unit=A  v2_specify=off  v2_priority=None  v2=0 V  v2_nominal_specify=off  v2_nominal_value=1  v2_nominal_unit=V
  Inductor : fl_lib/Electrical/Electrical Elements/Inductor  l=21e-6 H  r=1e-6 Ohm  g=0 1/Ohm  i_specify=off  i_priority=None  i=0 A  i_nominal_specify=off  i_nominal_value=1  i_nominal_unit=A  v_specify=off  v_priority=None  v=0 V  v_nominal_specify=off  v_nominal_value=1  v_nominal_unit=V  i_L_specify=off  i_L_priority=High  i_L=0 A  i_L_nominal_specify=off  i_L_nominal_value=1  i_L_nominal_unit=A
  PS-Simulink Converter2 : nesl_utility/PS-Simulink Converter  PhysicalDomain=network_engine_domain  SubClassName=ps_output  LeftPortType=input  RightPortType=output  PseudoPeriodic=off  Frequencies=[]  VectorFormat=inherit  Unit=inherit  AffineConversion=off
  S1 : Subsystem
      settings: PortSchema="{\"entries\":[{\"content\":{\"sides\":[{\"content\":{\"connectorIds\":[\"In1\"]},\"type\":\"ConnectorPlacement.EquallySpacedRectSide\",\"uuid\":\"4868c43b-8f86-4e2f-a4da-367c2e17d6e4\"},{\"content\":{\"side\":\"RIGHT\"},\"type\":\"ConnectorPlacement.EquallySpacedRectSide\",\"uuid\":\"ebe9b5ec-833b-4a08-98e5-ff684cd7afcb\"},{\"content\":{\"connectorIds\":[\"LConn1\"],\"side\":\"TOP\"},\"type\":\"ConnectorPlacement.EquallySpacedRectSide\",\"uuid\":\"c72df866-8baa-41a8-9bb1-42a4a1fdee71\"},{\"content\":{\"connectorIds\":[\"RConn1\"],\"side\":\"BOTTOM\"},\"type\":\"ConnectorPlacement.EquallySpacedRectSide\",\"uuid\":\"3a9867c5-1563-48cb-a4f4-92deec85fd3d\"}]},\"type\":\"ConnectorPlacement.EquallySpacedConnector\",\"uuid\":\"206e0d7b-1d35-45e7-9c4c-8a6f9fe9dc79\"}],\"packageUris\":[\"http://schema.mathworks.com/mf0/Connector/R2020b\"],\"version\":\"1.0\"}"
  S2 : Subsystem
      settings: PortSchema="{\"entries\":[{\"content\":{\"sides\":[{\"content\":{\"connectorIds\":[\"In1\"]},\"type\":\"ConnectorPlacement.EquallySpacedRectSide\",\"uuid\":\"4868c43b-8f86-4e2f-a4da-367c2e17d6e4\"},{\"content\":{\"side\":\"RIGHT\"},\"type\":\"ConnectorPlacement.EquallySpacedRectSide\",\"uuid\":\"ebe9b5ec-833b-4a08-98e5-ff684cd7afcb\"},{\"content\":{\"connectorIds\":[\"LConn1\"],\"side\":\"TOP\"},\"type\":\"ConnectorPlacement.EquallySpacedRectSide\",\"uuid\":\"c72df866-8baa-41a8-9bb1-42a4a1fdee71\"},{\"content\":{\"connectorIds\":[\"RConn1\"],\"side\":\"BOTTOM\"},\"type\":\"ConnectorPlacement.EquallySpacedRectSide\",\"uuid\":\"3a9867c5-1563-48cb-a4f4-92deec85fd3d\"}]},\"type\":\"ConnectorPlacement.EquallySpacedConnector\",\"uuid\":\"206e0d7b-1d35-45e7-9c4c-8a6f9fe9dc79\"}],\"packageUris\":[\"http://schema.mathworks.com/mf0/Connector/R2020b\"],\"version\":\"1.0\"}"
  S3 : Subsystem
      settings: PortSchema="{\"entries\":[{\"content\":{\"sides\":[{\"content\":{\"connectorIds\":[\"In1\"]},\"type\":\"ConnectorPlacement.EquallySpacedRectSide\",\"uuid\":\"4868c43b-8f86-4e2f-a4da-367c2e17d6e4\"},{\"content\":{\"side\":\"RIGHT\"},\"type\":\"ConnectorPlacement.EquallySpacedRectSide\",\"uuid\":\"ebe9b5ec-833b-4a08-98e5-ff684cd7afcb\"},{\"content\":{\"connectorIds\":[\"LConn1\"],\"side\":\"TOP\"},\"type\":\"ConnectorPlacement.EquallySpacedRectSide\",\"uuid\":\"c72df866-8baa-41a8-9bb1-42a4a1fdee71\"},{\"content\":{\"connectorIds\":[\"RConn1\"],\"side\":\"BOTTOM\"},\"type\":\"ConnectorPlacement.EquallySpacedRectSide\",\"uuid\":\"3a9867c5-1563-48cb-a4f4-92deec85fd3d\"}]},\"type\":\"ConnectorPlacement.EquallySpacedConnector\",\"uuid\":\"206e0d7b-1d35-45e7-9c4c-8a6f9fe9dc79\"}],\"packageUris\":[\"http://schema.mathworks.com/mf0/Connector/R2020b\"],\"version\":\"1.0\"}"
  S4 : Subsystem
      settings: PortSchema="{\"entries\":[{\"content\":{\"sides\":[{\"content\":{\"connectorIds\":[\"In1\"]},\"type\":\"ConnectorPlacement.EquallySpacedRectSide\",\"uuid\":\"4868c43b-8f86-4e2f-a4da-367c2e17d6e4\"},{\"content\":{\"side\":\"RIGHT\"},\"type\":\"ConnectorPlacement.EquallySpacedRectSide\",\"uuid\":\"ebe9b5ec-833b-4a08-98e5-ff684cd7afcb\"},{\"content\":{\"connectorIds\":[\"LConn1\"],\"side\":\"TOP\"},\"type\":\"ConnectorPlacement.EquallySpacedRectSide\",\"uuid\":\"c72df866-8baa-41a8-9bb1-42a4a1fdee71\"},{\"content\":{\"connectorIds\":[\"RConn1\"],\"side\":\"BOTTOM\"},\"type\":\"ConnectorPlacement.EquallySpacedRectSide\",\"uuid\":\"3a9867c5-1563-48cb-a4f4-92deec85fd3d\"}]},\"type\":\"ConnectorPlacement.EquallySpacedConnector\",\"uuid\":\"206e0d7b-1d35-45e7-9c4c-8a6f9fe9dc79\"}],\"packageUris\":[\"http://schema.mathworks.com/mf0/Connector/R2020b\"],\"version\":\"1.0\"}"
  Unit Delay1 : UnitDelay  SampleTime=-1
  +1 : PMIOPort  Side=Left
  -1 : PMIOPort  Port=2  Side=Left
  +2 : PMIOPort  Port=3  Side=Right
  -2 : PMIOPort  Port=4  Side=Right
  tag scope: I_charging2=global
  wires:
  [Ss_a_u2] -> Data Type Conversion2/1
  [Ss_a_u2] -> Data Type Conversion1/1
  PS-Simulink Converter2/1 -> Unit Delay1/1
  [Ss_a_l2] -> Data Type Conversion5/1
  [Ss_a_l2] -> Data Type Conversion3/1
  Data Type Conversion5/1 -> S3/1(g)
  Data Type Conversion1/1 -> S4/1(g)
  Data Type Conversion2/1 -> S1/1(g)
  Data Type Conversion3/1 -> S2/1(g)
  Unit Delay1/1 -> [I_charging2]
  connections:
  Current Sensor/RConn2 -- +2/RConn1
  -1/RConn1 -- S2/RConn1 -- S4/RConn1
  Ideal Transformer/RConn1 -- Diode1/RConn1 -- Diode13/LConn1
  Current Sensor/RConn1 -- PS-Simulink Converter2/LConn1
  Ideal Transformer/LConn1 -- Capacitor2/RConn1
  -2/RConn1 -- Diode3/LConn1 -- Diode1/LConn1 -- Capacitor3/RConn1
  S4/LConn1 -- Capacitor2/LConn1 -- S3/RConn1
  +1/RConn1 -- S1/LConn1 -- S3/LConn1
  Ideal Transformer/RConn2 -- Diode3/RConn1 -- Diode2/LConn1
  Inductor/RConn1 -- Ideal Transformer/LConn2
  Current Sensor/LConn1 -- Diode2/RConn1 -- Diode13/RConn1 -- Capacitor3/LConn1
  S1/RConn1 -- Inductor/LConn1 -- S2/LConn1

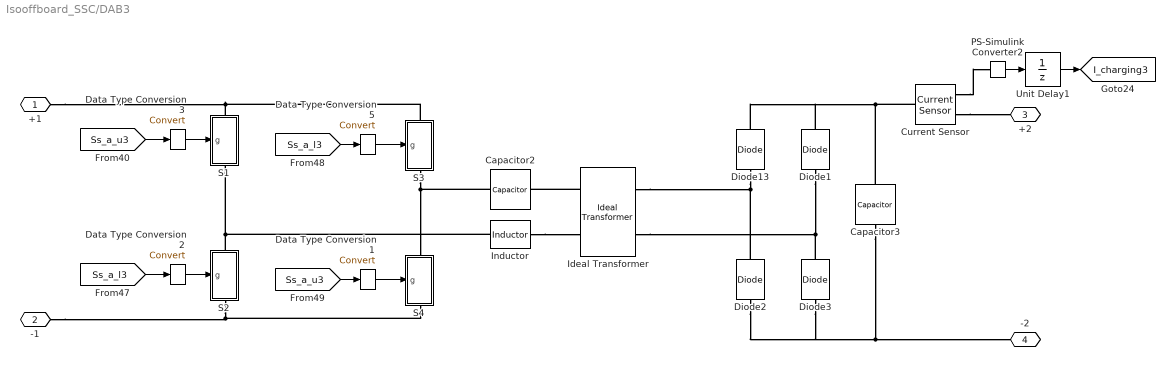
== system Isooffboard_SSC/DAB3 ==
  Capacitor2 : fl_lib/Electrical/Electrical Elements/Capacitor  c=110e-9 F  r=1e-6 Ohm  g=0 1/Ohm  i_specify=off  i_priority=None  i=0 A  i_nominal_specify=off  i_nominal_value=1  i_nominal_unit=A  v_specify=off  v_priority=None  v=0 V  v_nominal_specify=off  v_nominal_value=1  v_nominal_unit=V  vc_specify=off  vc_priority=High  vc=0 V  vc_nominal_specify=off  vc_nominal_value=1  vc_nominal_unit=V
  Capacitor3 : fl_lib/Electrical/Electrical Elements/Capacitor  c=500e-6 F  r=0 Ohm  g=0 1/Ohm  i_specify=off  i_priority=None  i=0 A  i_nominal_specify=off  i_nominal_value=1  i_nominal_unit=A  v_specify=off  v_priority=None  v=0 V  v_nominal_specify=off  v_nominal_value=1  v_nominal_unit=V  vc_specify=off  vc_priority=High  vc=0 V  vc_nominal_specify=off  vc_nominal_value=1  vc_nominal_unit=V
  Current Sensor : fl_lib/Electrical/Electrical Sensors/Current Sensor
  Data Type Conversion{1..3,5} (4 alike) : DataTypeConversion  SaturateOnIntegerOverflow=off  RndMeth=Floor
  Diode{1..3,13} (4 alike) : fl_lib/Electrical/Electrical Elements/Diode  Vf=0.8 V  Ron=0.001 Ohm  Goff=1/500 1/Ohm  i_specify=off  i_priority=None  i=0 A  i_nominal_specify=off  i_nominal_value=1  i_nominal_unit=A  v_specify=off  v_priority=None  v=0 V  v_nominal_specify=off  v_nominal_value=1  v_nominal_unit=V
  Ideal Transformer : fl_lib/Electrical/Electrical Elements/Ideal Transformer  n=1  i1_specify=off  i1_priority=None  i1=0 A  i1_nominal_specify=off  i1_nominal_value=1  i1_nominal_unit=A  v1_specify=off  v1_priority=None  v1=0 V  v1_nominal_specify=off  v1_nominal_value=1  v1_nominal_unit=V  i2_specify=off  i2_priority=None  i2=0 A  i2_nominal_specify=off  i2_nominal_value=1  i2_nominal_unit=A  v2_specify=off  v2_priority=None  v2=0 V  v2_nominal_specify=off  v2_nominal_value=1  v2_nominal_unit=V
  Inductor : fl_lib/Electrical/Electrical Elements/Inductor  l=21e-6 H  r=1e-6 Ohm  g=0 1/Ohm  i_specify=off  i_priority=None  i=0 A  i_nominal_specify=off  i_nominal_value=1  i_nominal_unit=A  v_specify=off  v_priority=None  v=0 V  v_nominal_specify=off  v_nominal_value=1  v_nominal_unit=V  i_L_specify=off  i_L_priority=High  i_L=0 A  i_L_nominal_specify=off  i_L_nominal_value=1  i_L_nominal_unit=A
  PS-Simulink Converter2 : nesl_utility/PS-Simulink Converter  PhysicalDomain=network_engine_domain  SubClassName=ps_output  LeftPortType=input  RightPortType=output  PseudoPeriodic=off  Frequencies=[]  VectorFormat=inherit  Unit=inherit  AffineConversion=off
  S1 : Subsystem
      settings: PortSchema="{\"entries\":[{\"content\":{\"sides\":[{\"content\":{\"connectorIds\":[\"In1\"]},\"type\":\"ConnectorPlacement.EquallySpacedRectSide\",\"uuid\":\"4868c43b-8f86-4e2f-a4da-367c2e17d6e4\"},{\"content\":{\"side\":\"RIGHT\"},\"type\":\"ConnectorPlacement.EquallySpacedRectSide\",\"uuid\":\"ebe9b5ec-833b-4a08-98e5-ff684cd7afcb\"},{\"content\":{\"connectorIds\":[\"LConn1\"],\"side\":\"TOP\"},\"type\":\"ConnectorPlacement.EquallySpacedRectSide\",\"uuid\":\"c72df866-8baa-41a8-9bb1-42a4a1fdee71\"},{\"content\":{\"connectorIds\":[\"RConn1\"],\"side\":\"BOTTOM\"},\"type\":\"ConnectorPlacement.EquallySpacedRectSide\",\"uuid\":\"3a9867c5-1563-48cb-a4f4-92deec85fd3d\"}]},\"type\":\"ConnectorPlacement.EquallySpacedConnector\",\"uuid\":\"206e0d7b-1d35-45e7-9c4c-8a6f9fe9dc79\"}],\"packageUris\":[\"http://schema.mathworks.com/mf0/Connector/R2020b\"],\"version\":\"1.0\"}"
  S2 : Subsystem
      settings: PortSchema="{\"entries\":[{\"content\":{\"sides\":[{\"content\":{\"connectorIds\":[\"In1\"]},\"type\":\"ConnectorPlacement.EquallySpacedRectSide\",\"uuid\":\"4868c43b-8f86-4e2f-a4da-367c2e17d6e4\"},{\"content\":{\"side\":\"RIGHT\"},\"type\":\"ConnectorPlacement.EquallySpacedRectSide\",\"uuid\":\"ebe9b5ec-833b-4a08-98e5-ff684cd7afcb\"},{\"content\":{\"connectorIds\":[\"LConn1\"],\"side\":\"TOP\"},\"type\":\"ConnectorPlacement.EquallySpacedRectSide\",\"uuid\":\"c72df866-8baa-41a8-9bb1-42a4a1fdee71\"},{\"content\":{\"connectorIds\":[\"RConn1\"],\"side\":\"BOTTOM\"},\"type\":\"ConnectorPlacement.EquallySpacedRectSide\",\"uuid\":\"3a9867c5-1563-48cb-a4f4-92deec85fd3d\"}]},\"type\":\"ConnectorPlacement.EquallySpacedConnector\",\"uuid\":\"206e0d7b-1d35-45e7-9c4c-8a6f9fe9dc79\"}],\"packageUris\":[\"http://schema.mathworks.com/mf0/Connector/R2020b\"],\"version\":\"1.0\"}"
  S3 : Subsystem
      settings: PortSchema="{\"entries\":[{\"content\":{\"sides\":[{\"content\":{\"connectorIds\":[\"In1\"]},\"type\":\"ConnectorPlacement.EquallySpacedRectSide\",\"uuid\":\"4868c43b-8f86-4e2f-a4da-367c2e17d6e4\"},{\"content\":{\"side\":\"RIGHT\"},\"type\":\"ConnectorPlacement.EquallySpacedRectSide\",\"uuid\":\"ebe9b5ec-833b-4a08-98e5-ff684cd7afcb\"},{\"content\":{\"connectorIds\":[\"LConn1\"],\"side\":\"TOP\"},\"type\":\"ConnectorPlacement.EquallySpacedRectSide\",\"uuid\":\"c72df866-8baa-41a8-9bb1-42a4a1fdee71\"},{\"content\":{\"connectorIds\":[\"RConn1\"],\"side\":\"BOTTOM\"},\"type\":\"ConnectorPlacement.EquallySpacedRectSide\",\"uuid\":\"3a9867c5-1563-48cb-a4f4-92deec85fd3d\"}]},\"type\":\"ConnectorPlacement.EquallySpacedConnector\",\"uuid\":\"206e0d7b-1d35-45e7-9c4c-8a6f9fe9dc79\"}],\"packageUris\":[\"http://schema.mathworks.com/mf0/Connector/R2020b\"],\"version\":\"1.0\"}"
  S4 : Subsystem
      settings: PortSchema="{\"entries\":[{\"content\":{\"sides\":[{\"content\":{\"connectorIds\":[\"In1\"]},\"type\":\"ConnectorPlacement.EquallySpacedRectSide\",\"uuid\":\"4868c43b-8f86-4e2f-a4da-367c2e17d6e4\"},{\"content\":{\"side\":\"RIGHT\"},\"type\":\"ConnectorPlacement.EquallySpacedRectSide\",\"uuid\":\"ebe9b5ec-833b-4a08-98e5-ff684cd7afcb\"},{\"content\":{\"connectorIds\":[\"LConn1\"],\"side\":\"TOP\"},\"type\":\"ConnectorPlacement.EquallySpacedRectSide\",\"uuid\":\"c72df866-8baa-41a8-9bb1-42a4a1fdee71\"},{\"content\":{\"connectorIds\":[\"RConn1\"],\"side\":\"BOTTOM\"},\"type\":\"ConnectorPlacement.EquallySpacedRectSide\",\"uuid\":\"3a9867c5-1563-48cb-a4f4-92deec85fd3d\"}]},\"type\":\"ConnectorPlacement.EquallySpacedConnector\",\"uuid\":\"206e0d7b-1d35-45e7-9c4c-8a6f9fe9dc79\"}],\"packageUris\":[\"http://schema.mathworks.com/mf0/Connector/R2020b\"],\"version\":\"1.0\"}"
  Unit Delay1 : UnitDelay  SampleTime=-1
  +1 : PMIOPort  Side=Left
  -1 : PMIOPort  Port=2  Side=Left
  +2 : PMIOPort  Port=3  Side=Right
  -2 : PMIOPort  Port=4  Side=Right
  tag scope: I_charging3=global
  wires:
  [Ss_a_l3] -> Data Type Conversion2/1
  [Ss_a_l3] -> Data Type Conversion5/1
  PS-Simulink Converter2/1 -> Unit Delay1/1
  [Ss_a_u3] -> Data Type Conversion1/1
  [Ss_a_u3] -> Data Type Conversion3/1
  Data Type Conversion5/1 -> S3/1(g)
  Data Type Conversion1/1 -> S4/1(g)
  Data Type Conversion2/1 -> S2/1(g)
  Data Type Conversion3/1 -> S1/1(g)
  Unit Delay1/1 -> [I_charging3]
  connections:
  S2/LConn1 -- Inductor/LConn1 -- S1/RConn1
  Capacitor3/LConn1 -- Diode1/RConn1 -- Diode13/RConn1 -- Current Sensor/LConn1
  Inductor/RConn1 -- Ideal Transformer/LConn2
  Ideal Transformer/RConn2 -- Diode3/RConn1 -- Diode1/LConn1
  S3/LConn1 -- S1/LConn1 -- +1/RConn1
  S3/RConn1 -- Capacitor2/LConn1 -- S4/LConn1
  Capacitor3/RConn1 -- Diode3/LConn1 -- Diode2/LConn1 -- -2/RConn1
  Ideal Transformer/LConn1 -- Capacitor2/RConn1
  Current Sensor/RConn1 -- PS-Simulink Converter2/LConn1
  Ideal Transformer/RConn1 -- Diode2/RConn1 -- Diode13/LConn1
  S4/RConn1 -- S2/RConn1 -- -1/RConn1
  Current Sensor/RConn2 -- +2/RConn1
